simulink model "vocoder"  (R2025b)
settings: Solver=FixedStepDiscrete  StartTime=0.0  StopTime=inf  FixedStep=128/48000  RelTol=1e-3
undefined symbols (not defined in the file): Attack_rt, Mix_rt, Release_rt
settings Model: Creator=linogarciamorales  LastModifiedBy=linogarciamorales
settings OptimizationCC: EnhancedBackFolding=on  PassReuseOutputArgsAs=Individual arguments  ZeroExternalMemoryAtStartup=off  ZeroInternalMemoryAtStartup=off  OptimizeBlockOrder=speed  DifferentSizesBufferReuse=on  OptimizationCustomize=off  EfficientTunableParamExpr=on
settings DebuggingCC: ParameterTunabilityLossMsg=error
settings SFSimCC: MATLABDynamicMemAlloc=off
settings RTWCC: SystemTargetFile=ert.tlc  GenCodeOnly=on  TemplateMakefile=ert_default_tmf  Description=Embedded Coder
settings CodeAppCC: ForceParamTrailComments=on  IgnoreCustomStorageClasses=off  OperatorAnnotations=on  SimulinkDataObjDesc=on  SFDataObjDesc=on  InsertBlockDesc=on
settings ERTTargetCC: InlinedParameterPlacement=Hierarchical  ERTCustomFileTemplate=example_file_process.tlc  TargetLangStandard=C99 (ISO)  GenerateSampleERTMain=on  SupportNonInlinedSFcns=on  SupportVariableSizeSignals=on

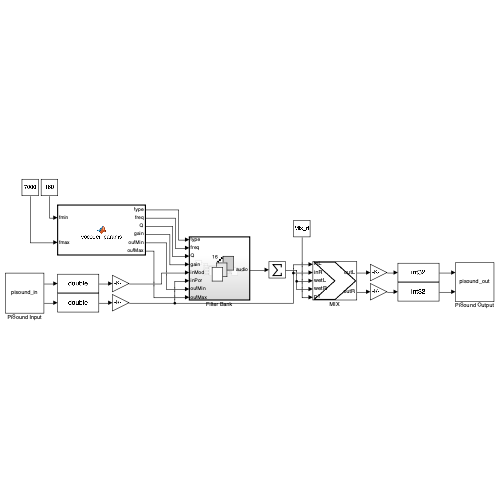
[thumbnail: Simulink's stored preview of the top-level diagram]
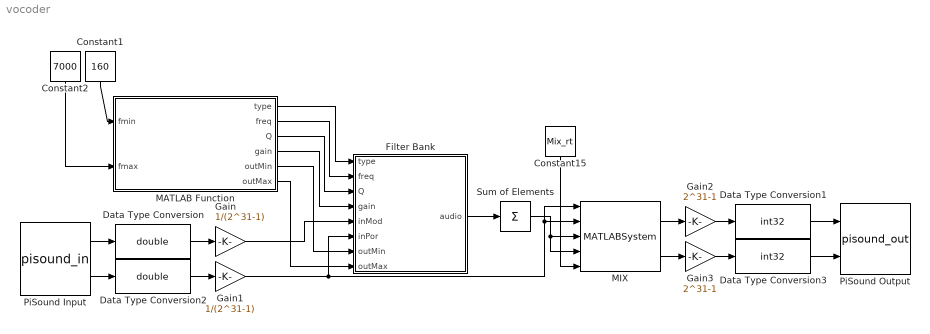
== system vocoder ==
  Constant1 : Constant  Value=160  OutDataTypeStr=double
  Constant15 : Constant  Value=Mix_rt  OutDataTypeStr=double
  Constant2 : Constant  Value=7000  OutDataTypeStr=double
  Data Type Conversion : DataTypeConversion  OutDataTypeStr=double  SaturateOnIntegerOverflow=off  RndMeth=Floor
  Data Type Conversion1 : DataTypeConversion  OutDataTypeStr=int32  SaturateOnIntegerOverflow=off  RndMeth=Floor
  Data Type Conversion2 : DataTypeConversion  OutDataTypeStr=double  SaturateOnIntegerOverflow=off  RndMeth=Floor
  Data Type Conversion3 : DataTypeConversion  OutDataTypeStr=int32  SaturateOnIntegerOverflow=off  RndMeth=Floor
  Filter Bank : Subsystem  TreatAsAtomicUnit=on
  Gain : Gain  Gain=1/(2^31-1)
  Gain1 : Gain  Gain=1/(2^31-1)
  Gain2 : Gain  Gain=2^31-1
  Gain3 : Gain  Gain=2^31-1
  MATLAB Function : MATLAB Function  TreatAsAtomicUnit=on
  MIX : MATLABSystem  System=mix_sys  N=128  Fs=48000  Mode=uint8( 0 )  SmoothTime=0.01  IndepInDB=false  SimulateUsing=Code generation
      mask Type: mix_sys
  PiSound Input : S-Function  FunctionName=pisound_in  Parameters=48000, 128, 0  SFunctionDeploymentMode=off  EnableBusSupport=off
  PiSound Output : S-Function  FunctionName=pisound_out  Parameters=48000, 128, 0  SFunctionDeploymentMode=off  EnableBusSupport=off
  Sum of Elements : Sum  Inputs=+  CollapseMode=Specified dimension  CollapseDim=2
  wires:
  PiSound Input/1 -> Data Type Conversion/1
  PiSound Input/2 -> Data Type Conversion2/1
  Data Type Conversion1/1 -> PiSound Output/1
  Data Type Conversion3/1 -> PiSound Output/2
  Gain2/1 -> Data Type Conversion1/1
  Gain3/1 -> Data Type Conversion3/1
  Data Type Conversion/1 -> Gain/1
  Data Type Conversion2/1 -> Gain1/1
  MIX/1 -> Gain2/1
  MIX/2 -> Gain3/1
  Constant15/1 -> MIX/5
  MATLAB Function/1(type) -> Filter Bank/1(type)
  MATLAB Function/2(freq) -> Filter Bank/2(freq)
  MATLAB Function/3(Q) -> Filter Bank/3(Q)
  MATLAB Function/4(gain) -> Filter Bank/4(gain)
  Gain/1 -> Filter Bank/5(inMod)
  Constant1/1 -> MATLAB Function/1(fmin)
  Constant2/1 -> MATLAB Function/2(fmax)
  Gain1/1 -> MIX/1, MIX/2, Filter Bank/6(inPor)
  Sum of Elements/1 -> MIX/4, MIX/3
  MATLAB Function/5(outMin) -> Filter Bank/7(outMin)
  MATLAB Function/6(outMax) -> Filter Bank/8(outMax)
  Filter Bank/1(audio) -> Sum of Elements/1

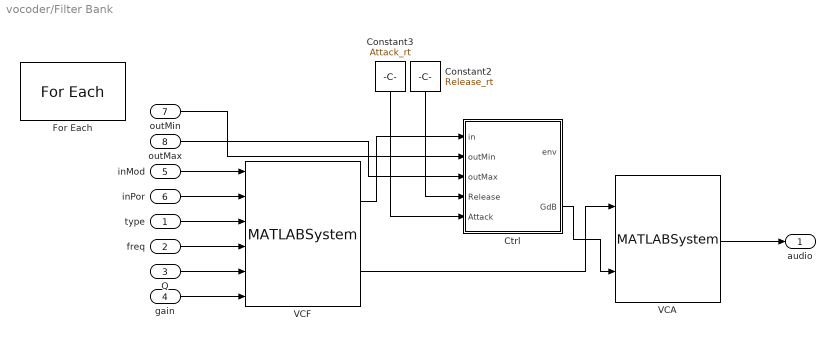
== system vocoder/Filter Bank ==
  type : Inport  Partition=on  PartitionDimension=1  PartitionWidth=1  PartitionOffset=0
  freq : Inport  Port=2  Partition=on  PartitionDimension=1  PartitionWidth=1  PartitionOffset=0
  Q : Inport  Port=3  Partition=on  PartitionDimension=1  PartitionWidth=1  PartitionOffset=0
  gain : Inport  Port=4  Partition=on  PartitionDimension=1  PartitionWidth=1  PartitionOffset=0
  inMod : Inport  Tag=inLmod  Port=5
  inPor : Inport  Port=6
  outMin : Inport  Port=7  Partition=on  PartitionDimension=1  PartitionWidth=1  PartitionOffset=0
  outMax : Inport  Port=8  Partition=on  PartitionDimension=1  PartitionWidth=1  PartitionOffset=0
  Constant2 : Constant  Value=Release_rt  OutDataTypeStr=double
  Constant3 : Constant  Value=Attack_rt  OutDataTypeStr=double
  Ctrl : Subsystem
  For Each : ForEach  DisableCoverage=on  ShowIterationIndex=on
  VCA : MATLABSystem  System=vca_mono_sys  N=128  Fs=48000  bypass=uint8(0)  Mode=uint8(1)  ForceGainEnable=uint8(0)  ForceGainValue=-20  SimulateUsing=Code generation
      mask Type: vca_mono_sys
  VCF : MATLABSystem  System=vcf_sys  N=128  Fs=48000  bypass=uint8(0)  SimulateUsing=Code generation
      mask Type: vcf_sys
  audio : Outport  OutDataTypeStr=double  ConcatenationDimension=2
  wires:
  VCF/1 -> Ctrl/1(in)
  inPor/1 -> VCF/2
  type/1 -> VCF/3
  freq/1 -> VCF/4
  Q/1 -> VCF/5
  gain/1 -> VCF/6
  Constant2/1 -> Ctrl/4(Release)
  Constant3/1 -> Ctrl/5(Attack)
  outMin/1 -> Ctrl/2(outMin)
  outMax/1 -> Ctrl/3(outMax)
  VCF/2 -> VCA/1
  inMod/1 -> VCF/1
  VCA/1 -> audio/1
  Ctrl/2(GdB) -> VCA/2

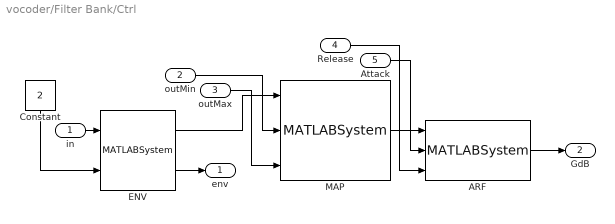
== system vocoder/Filter Bank/Ctrl ==
  in : Inport
  outMin : Inport  Port=2
  outMax : Inport  Port=3
  Release : Inport  Port=4
  Attack : Inport  Port=5
  ARF : MATLABSystem  System=arf_sys  N=128  Fs=48000  bypass=uint8(0)  SimulateUsing=Code generation
      mask Type: arf_sys
  Constant : Constant  Value=2  OutDataTypeStr=uint8
  ENV : MATLABSystem  System=env_mono_sys  N=128  Fs=48000  ModeDefault=uint8(2)  Eps=1e-12  TauRMS=0.02  SimulateUsing=Code generation
      mask Type: env_mono_sys
  MAP : MATLABSystem  System=map_sys  bypass=uint8(0)  Mode=uint8(1)  Threshold=-45  Slope=2  SimulateUsing=Code generation  Offset=22
      mask Type: map_sys
  env : Outport
  GdB : Outport  Port=2
  wires:
  Constant/1 -> ENV/2
  in/1 -> ENV/1
  Release/1 -> ARF/3
  Attack/1 -> ARF/2
  MAP/1 -> ARF/1
  ENV/1 -> MAP/1
  outMin/1 -> MAP/2
  outMax/1 -> MAP/3
  ENV/2 -> env/1
  ARF/1 -> GdB/1

== matlab function vocoder/MATLAB Function ==
  data: type output; fmin input; fmax input; freq output; Q output; gain output; outMin output; outMax output
function [type,freq,Q,gain,outMin,outMax] = vocoder_params(fmin,fmax)
%#codegen
  K = int32(16);
  [type,freq,Q,gain] = fb_params(fmin,fmax,K);
  [outMin,outMax] = ctrl_params_from_freq(freq,K);
  type = type(1:K);
  freq = freq(1:K);
  Q    = Q(1:K);
  gain = gain(1:K);
end
